simulink model "digital_twin_irrigation"  (R2025b)
settings: Solver=FixedStepDiscrete  StartTime=0.0  StopTime=60  FixedStep=1  RelTol=1e-3
settings Model: LastModifiedBy=chenn

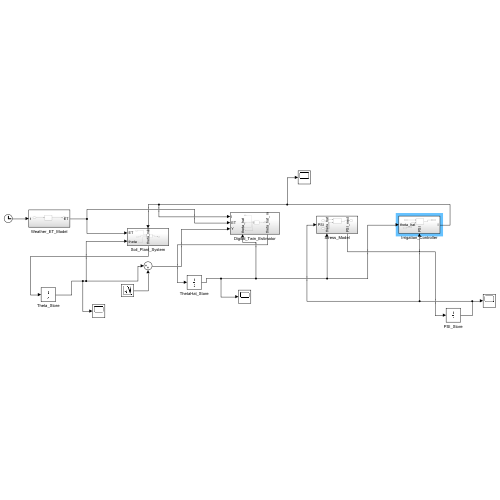
[thumbnail: Simulink's stored preview of the top-level diagram]
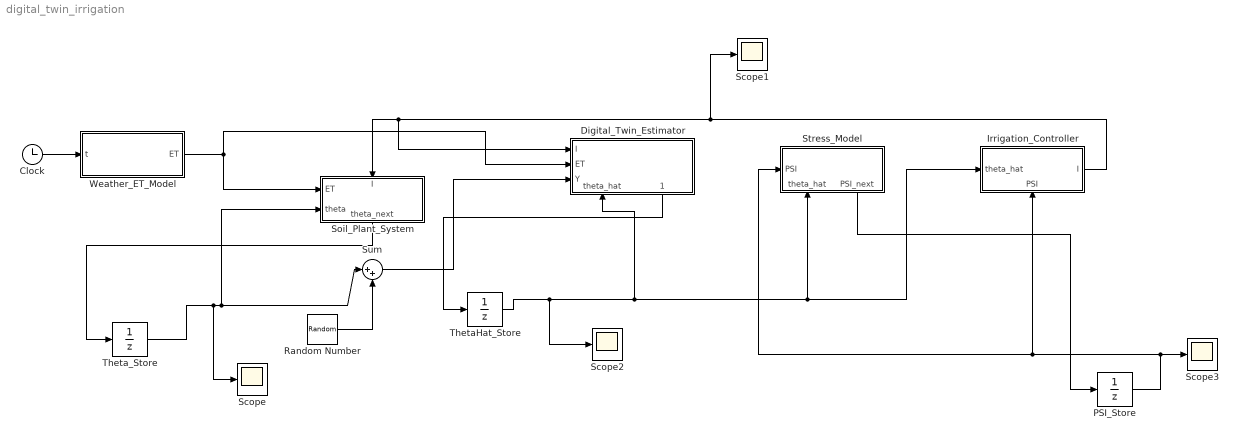
== system digital_twin_irrigation ==
  Clock : Clock
  Digital_Twin_Estimator : Subsystem
      settings: PortSchema="{\"entries\":[{\"content\":{\"sides\":[{\"content\":{\"connectorIds\":[\"In1\",\"In2\",\"In3\"]},\"type\":\"ConnectorPlacement.EquallySpacedRectSide\",\"uuid\":\"021b26ad-0b79-40cd-9053-9fc75d1ca9f8\"},{\"content\":{\"side\":\"RIGHT\"},\"type\":\"ConnectorPlacement.EquallySpacedRectSide\",\"uuid\":\"689f36c4-e74d-44a6-8ab8-420f648872b2\"},{\"content\":{\"side\":\"TOP\"},\"type\":\"ConnectorPlacement.EquallySpacedRectSide\",\"uuid\":\"8878a85e-e00f-4519-97d4-2908e3e4ef62\"},{\"content\":{\"connectorIds\":[\"In4\",\"Out1\"],\"side\":\"BOTTOM\"},\"type\":\"ConnectorPlacement.EquallySpacedRectSide\",\"uuid\":\"b7a47bf2-3c5e-48b1-b7d2-e71432755ad3\"}]},\"type\":\"ConnectorPlacement.EquallySpacedConnector\",\"uuid\":\"37a8765f-1bc4-485a-9681-3e0bccf9abb0\"}],\"packageUris\":[\"http://schema.mathworks.com/mf0/Connector/R2020b\"],\"version\":\"1.0\"}"
  Irrigation_Controller : Subsystem
      settings: PortSchema="{\"entries\":[{\"content\":{\"sides\":[{\"content\":{\"connectorIds\":[\"In1\"]},\"type\":\"ConnectorPlacement.EquallySpacedRectSide\",\"uuid\":\"b9e01bb4-6d94-4b22-9a59-85253c67ab33\"},{\"content\":{\"connectorIds\":[\"Out1\"],\"side\":\"RIGHT\"},\"type\":\"ConnectorPlacement.EquallySpacedRectSide\",\"uuid\":\"6b15fbcb-21d0-435f-ad64-e1ac440dabd5\"},{\"content\":{\"side\":\"TOP\"},\"type\":\"ConnectorPlacement.EquallySpacedRectSide\",\"uuid\":\"ab4925f1-9e63-43e6-ad3f-15721e695062\"},{\"content\":{\"connectorIds\":[\"In2\"],\"side\":\"BOTTOM\"},\"type\":\"ConnectorPlacement.EquallySpacedRectSide\",\"uuid\":\"feb922c7-8166-4d1d-91a7-db938aee2250\"}]},\"type\":\"ConnectorPlacement.EquallySpacedConnector\",\"uuid\":\"f39a5bc5-648a-469d-aa5c-161580002f84\"}],\"packageUris\":[\"http://schema.mathworks.com/mf0/Connector/R2020b\"],\"version\":\"1.0\"}"
  PSI_Store : UnitDelay  HasFrameUpgradeWarning=on
  Random Number : RandomNumber  Variance=0.0001  SampleTime=1
  Scope{,1..3} (4 alike) : Scope
      Scope settings: ActiveDisplayYMinimum=-6.1750548747831466  ActiveDisplayYMaximum=0.96389498608701618
      Scope1 settings: ActiveDisplayYMinimum=-0.0012499999999999998  ActiveDisplayYMaximum=0.01125
      Scope2 settings: ActiveDisplayYMinimum=-6.1701666378085669  ActiveDisplayYMaximum=0.96335184864539625  DataLoggingVariableName=ScopeData2
      Scope3 settings: ActiveDisplayYMinimum=-89.72465317413355  ActiveDisplayYMaximum=807.52187856720207  DataLoggingVariableName=ScopeData3
  Soil_Plant_System : Subsystem
      settings: PortSchema="{\"entries\":[{\"content\":{\"sides\":[{\"content\":{\"connectorIds\":[\"In1\",\"In2\"]},\"type\":\"ConnectorPlacement.EquallySpacedRectSide\",\"uuid\":\"8f654530-0c93-4114-ad2e-d511ee5a27b3\"},{\"content\":{\"side\":\"RIGHT\"},\"type\":\"ConnectorPlacement.EquallySpacedRectSide\",\"uuid\":\"ca76a06a-9469-4024-8a55-2e4e9e50cbaf\"},{\"content\":{\"connectorIds\":[\"In3\"],\"side\":\"TOP\"},\"type\":\"ConnectorPlacement.EquallySpacedRectSide\",\"uuid\":\"322fa98c-f751-4ce5-9d90-2ca428b0a77c\"},{\"content\":{\"connectorIds\":[\"Out1\"],\"side\":\"BOTTOM\"},\"type\":\"ConnectorPlacement.EquallySpacedRectSide\",\"uuid\":\"c8719ea2-25f8-4e9d-8f40-ea37a36455ac\"}]},\"type\":\"ConnectorPlacement.EquallySpacedConnector\",\"uuid\":\"da260b04-30b3-451f-8318-2aeef5f4e0e4\"}],\"packageUris\":[\"http://schema.mathworks.com/mf0/Connector/R2020b\"],\"version\":\"1.0\"}"
  Stress_Model : Subsystem
      settings: PortSchema="{\"entries\":[{\"content\":{\"sides\":[{\"content\":{\"connectorIds\":[\"In1\"]},\"type\":\"ConnectorPlacement.EquallySpacedRectSide\",\"uuid\":\"b9e01bb4-6d94-4b22-9a59-85253c67ab33\"},{\"content\":{\"side\":\"RIGHT\"},\"type\":\"ConnectorPlacement.EquallySpacedRectSide\",\"uuid\":\"6b15fbcb-21d0-435f-ad64-e1ac440dabd5\"},{\"content\":{\"side\":\"TOP\"},\"type\":\"ConnectorPlacement.EquallySpacedRectSide\",\"uuid\":\"ab4925f1-9e63-43e6-ad3f-15721e695062\"},{\"content\":{\"connectorIds\":[\"In2\",\"Out1\"],\"side\":\"BOTTOM\"},\"type\":\"ConnectorPlacement.EquallySpacedRectSide\",\"uuid\":\"1ab15dd7-0363-408a-8c3b-95fbb606d3c5\"}]},\"type\":\"ConnectorPlacement.EquallySpacedConnector\",\"uuid\":\"f39a5bc5-648a-469d-aa5c-161580002f84\"}],\"packageUris\":[\"http://schema.mathworks.com/mf0/Connector/R2020b\"],\"version\":\"1.0\"}"
  Sum : Sum  Inputs=|++
  ThetaHat_Store : UnitDelay  InitialCondition=0.25  HasFrameUpgradeWarning=on
  Theta_Store : UnitDelay  InitialCondition=0.25  HasFrameUpgradeWarning=on
  Weather_ET_Model : Subsystem
  wires:
  Clock/1 -> Weather_ET_Model/1(t)
  Weather_ET_Model/1(ET) -> Digital_Twin_Estimator/2(ET), Soil_Plant_System/1(ET)
  Random Number/1 -> Sum/2
  Sum/1 -> Digital_Twin_Estimator/3(Y)
  Irrigation_Controller/1(I) -> Scope1/1, Digital_Twin_Estimator/1(I), Soil_Plant_System/3(I)
  Theta_Store/1 -> Soil_Plant_System/2(theta), Sum/1, Scope/1
  Soil_Plant_System/1(theta_next) -> Theta_Store/1
  Digital_Twin_Estimator/1(theta_hat_next) -> ThetaHat_Store/1
  ThetaHat_Store/1 -> Scope2/1, Stress_Model/2(theta_hat), Irrigation_Controller/1(theta_hat), Digital_Twin_Estimator/4(theta_hat)
  PSI_Store/1 -> Scope3/1, Irrigation_Controller/2(PSI), Stress_Model/1(PSI)
  Stress_Model/1(PSI_next) -> PSI_Store/1

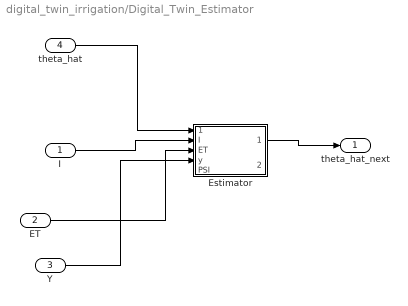
== system digital_twin_irrigation/Digital_Twin_Estimator ==
  I : Inport
  ET : Inport  Port=2
  Y : Inport  Port=3
  theta_hat : Inport  Port=4
  Estimator : MATLAB Function  TreatAsAtomicUnit=on
  theta_hat_next : Outport
  wires:
  theta_hat/1 -> Estimator/1(theta_hat)
  Estimator/1(theta_hat_next) -> theta_hat_next/1
  I/1 -> Estimator/2(I)
  ET/1 -> Estimator/3(ET)
  Y/1 -> Estimator/4(y)

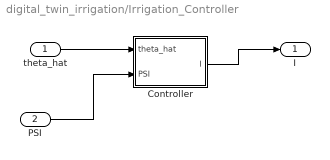
== system digital_twin_irrigation/Irrigation_Controller ==
  theta_hat : Inport
  PSI : Inport  Port=2
  Controller : MATLAB Function  TreatAsAtomicUnit=on
  I : Outport
  wires:
  theta_hat/1 -> Controller/1(theta_hat)
  PSI/1 -> Controller/2(PSI)
  Controller/1(I) -> I/1

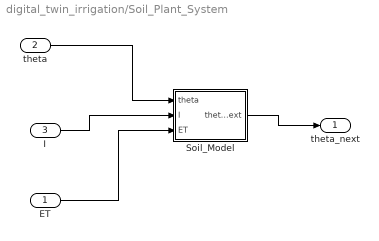
== system digital_twin_irrigation/Soil_Plant_System ==
  ET : Inport
  theta : Inport  Port=2
  I : Inport  Port=3
  Soil_Model : MATLAB Function  TreatAsAtomicUnit=on
  theta_next : Outport
  wires:
  theta/1 -> Soil_Model/1(theta)
  Soil_Model/1(theta_next) -> theta_next/1
  ET/1 -> Soil_Model/3(ET)
  I/1 -> Soil_Model/2(I)

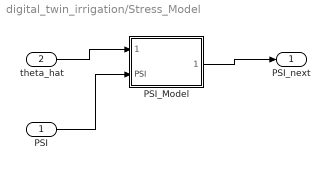
== system digital_twin_irrigation/Stress_Model ==
  PSI : Inport
  theta_hat : Inport  Port=2
  PSI_Model : MATLAB Function  TreatAsAtomicUnit=on
  PSI_next : Outport
  wires:
  theta_hat/1 -> PSI_Model/1(theta_hat)
  PSI_Model/1(PSI_next) -> PSI_next/1
  PSI/1 -> PSI_Model/2(PSI)

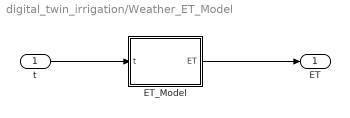
== system digital_twin_irrigation/Weather_ET_Model ==
  t : Inport
  ET_Model : MATLAB Function  TreatAsAtomicUnit=on
  ET : Outport
  wires:
  t/1 -> ET_Model/1(t)
  ET_Model/1(ET) -> ET/1

== matlab function digital_twin_irrigation/Soil_Plant_System/Soil_Model ==
  data: theta input; theta_next output; I input; ET input
function theta_next = Soil_Model(theta, I, ET)
params = parameters();
R = 0;
theta_next = soil_moisture_model(theta, I, ET, R, params);
theta_next = max(params.theta_wp, min(params.theta_fc, theta_next));

== matlab function digital_twin_irrigation/Weather_ET_Model/ET_Model ==
  data: t input; ET output
function ET = ET_Model(t)
params = parameters();
T_mean = 28 + 3*sin(2*pi*t/100);
T_max  = T_mean + 5;
T_min  = T_mean - 5;
delta_T = max(T_max - T_min, 0);
ET0 = 0.0023 * params.Ra * (T_mean + 17.8) * sqrt(delta_T);
ET  = ET0 / params.ET_scale;
ET  = max(0, ET);

== matlab function digital_twin_irrigation/Digital_Twin_Estimator/Estimator ==
  data: theta_hat input; theta_hat_next output; I input; ET input; y input; PSI input; PSI_next output
function [theta_hat_next, PSI_next] = Estimator(theta_hat, I, ET, y, PSI)
params = parameters();
persistent P
if isempty(P), P = 1; end
R_val = 0;
theta_pred = soil_moisture_model(theta_hat, I, ET, R_val, params);
P_pred = P + params.Q;
K = P_pred / (P_pred + params.R_noise);
theta_hat_next = theta_pred + K * (y - theta_pred);
theta_hat_next = max(params.theta_wp, min(params.theta_fc, theta_hat_next));
P = (1 - K) * P_pred;
PSI_next = plant_stress_model(PSI, theta_hat_next, params);

== matlab function digital_twin_irrigation/Stress_Model/PSI_Model ==
  data: theta_hat input; PSI_next output; PSI input
function PSI_next = PSI_Model(theta_hat, PSI)
params = parameters();
PSI_next = plant_stress_model(PSI, theta_hat, params);

== matlab function digital_twin_irrigation/Irrigation_Controller/Controller ==
  data: theta_hat input; I output; PSI input
function I = Controller(theta_hat, PSI)
params = parameters();
persistent last_irr iter
if isempty(last_irr)
    last_irr = -inf;
    iter = 1;
end
[I, last_irr] = digital_twin_controller(...
    theta_hat, PSI, iter, last_irr, params);
iter = iter + 1;
